simulink model "Boomerang_CoM_simulink"  (R2023a)
settings: Solver=ode4  StartTime=0.0  StopTime=t  FixedStep=dt  MaxStep=maxstep  MinStep=minstep
values from neighbouring files (symbols this model uses):
  c = 5e-2    (= 0.05)    [Boomerang4w_control.m]    (also in Boomerang_control_CoM.m = 0.0488; Boomerang_control_dihedral.m = 0.0488; Boomerang_control_gamma.m = 0.0488; Boomerang_control_pitch.m = 0.0488)
  CDdata = [x_CD, y_CD]    [Boomerang4w_control.m]    (also in Boomerang_control_CoM.m; Boomerang_control_dihedral.m; Boomerang_control_gamma.m; Boomerang_control_pitch.m)
  CLdata = [x_CL, y_CL]    [Boomerang4w_control.m]    (also in Boomerang_control_CoM.m; Boomerang_control_dihedral.m; Boomerang_control_gamma.m; Boomerang_control_pitch.m)
  CMdata = [x_CM, y_CM]    [Boomerang4w_control.m]    (also in Boomerang_control_CoM.m; Boomerang_control_dihedral.m; Boomerang_control_gamma.m; Boomerang_control_pitch.m)
  CoM_sat = 4e-2    (= 0.04)    [Boomerang4w_control.m]    (also in Boomerang_control_CoM.m = 0.02)
  Eul0 = [0; 0; 0]    [Boomerang4w_control.m]    (also in Boomerang_control_CoM.m; Boomerang_control_dihedral.m; Boomerang_control_gamma.m; Boomerang_control_pitch.m)
  g = 9.81    [Boomerang4w_control.m]    (also in Boomerang_control_CoM.m; Boomerang_control_dihedral.m; Boomerang_control_gamma.m; Boomerang_control_pitch.m)
  invTI0 = transpose(TI0)    [Boomerang4w_control.m]    (also in Boomerang_control_CoM.m; Boomerang_control_dihedral.m; Boomerang_control_gamma.m; Boomerang_control_pitch.m)
  J = J + (Ji(:,:,i))    [Boomerang4w_control.m]    (also in Boomerang_control_CoM.m = diag(diag(J)); Boomerang_control_dihedral.m = diag(diag(J)); Boomerang_control_gamma.m = diag(diag(J)); Boomerang_control_pitch.m = diag(diag(J)))
  Kd = 0.    (= 0)    [Boomerang4w_control.m]    (also in Boomerang_control_CoM.m; Boomerang_control_dihedral.m; Boomerang_control_gamma.m; Boomerang_control_pitch.m)
  Ki = 0.    (= 0)    [Boomerang4w_control.m]    (also in Boomerang_control_CoM.m; Boomerang_control_dihedral.m; Boomerang_control_gamma.m; Boomerang_control_pitch.m)
  Kp = .0    (= 0)    [Boomerang4w_control.m]    (also in Boomerang_control_CoM.m; Boomerang_control_dihedral.m; Boomerang_control_gamma.m; Boomerang_control_pitch.m)
  l_integrate = linspace(0,l_blade,n)    [Boomerang4w_control.m]    (also in Boomerang_control_CoM.m; Boomerang_control_dihedral.m; Boomerang_control_gamma.m; Boomerang_control_pitch.m)
  m = 200e-3    (= 0.2)    [Boomerang4w_control.m]    (also in Boomerang_control_CoM.m = 0.13; Boomerang_control_dihedral.m = 0.13; Boomerang_control_gamma.m = 0.13; Boomerang_control_pitch.m = 0.13)
  n = n + 1    (= 51)    [Boomerang4w_control.m]    (also in Boomerang_control_CoM.m; Boomerang_control_dihedral.m; Boomerang_control_gamma.m; Boomerang_control_pitch.m)
  nw = 4    [Boomerang4w_control.m]    (also in Boomerang_control_CoM.m = 2; Boomerang_control_dihedral.m = 2; Boomerang_control_gamma.m = 2; Boomerang_control_pitch.m = 2)
  omega0 = [0; 0; 10*pi*2]    [Boomerang4w_control.m]    (also in Boomerang_control_CoM.m; Boomerang_control_dihedral.m; Boomerang_control_gamma.m; Boomerang_control_pitch.m)
  PHI0 = deg2rad(PHI0)    [Boomerang4w_control.m]    (also in Boomerang_control_CoM.m; Boomerang_control_dihedral.m; Boomerang_control_gamma.m; Boomerang_control_pitch.m)
  PSI0 = deg2rad(PSI0)    [Boomerang4w_control.m]    (also in Boomerang_control_CoM.m; Boomerang_control_dihedral.m; Boomerang_control_gamma.m; Boomerang_control_pitch.m)
  R_pos0 = [0; 0; 1.5]    [Boomerang4w_control.m]    (also in Boomerang_control_CoM.m; Boomerang_control_dihedral.m; Boomerang_control_gamma.m; Boomerang_control_pitch.m)
  rate = 1    [Boomerang4w_control.m]    (also in Boomerang_control_CoM.m)
  rho = 1.22    [Boomerang4w_control.m]    (also in Boomerang_control_CoM.m; Boomerang_control_dihedral.m; Boomerang_control_gamma.m; Boomerang_control_pitch.m)
  S = pi*R^2    (= 0.196349540849)    [Boomerang4w_control.m]    (also in Boomerang_control_CoM.m = 0.228; Boomerang_control_dihedral.m = 0.228; Boomerang_control_gamma.m = 0.228; Boomerang_control_pitch.m = 0.228)
  THETA0 = deg2rad(THETA0)    [Boomerang4w_control.m]    (also in Boomerang_control_CoM.m; Boomerang_control_dihedral.m; Boomerang_control_gamma.m; Boomerang_control_pitch.m)
  thetaj = 25    [Boomerang4w_control.m]    (also in Boomerang_control_CoM.m = deg2rad(thetaj); Boomerang_control_dihedral.m = deg2rad(thetaj); Boomerang_control_gamma.m = deg2rad(thetaj); Boomerang_control_pitch.m = deg2rad(thetaj))
  TI0 = RI01*RI02*RI03    [Boomerang4w_control.m]    (also in Boomerang_control_CoM.m; Boomerang_control_dihedral.m; Boomerang_control_gamma.m; Boomerang_control_pitch.m)
  u0 = TI0*U0    [Boomerang4w_control.m]    (also in Boomerang_control_CoM.m; Boomerang_control_dihedral.m; Boomerang_control_gamma.m; Boomerang_control_pitch.m)
  v_wind = [-1; 0; 0]    [Boomerang4w_control.m]    (also in Boomerang_control_CoM.m = [0; 0; 0]; Boomerang_control_dihedral.m = [0; 0; 0]; Boomerang_control_gamma.m = [0; 0; 0]; Boomerang_control_pitch.m = [0; 0; 0])
  x_ac = zeros(3,nw)    [Boomerang4w_control.m]    (also in Boomerang_control_CoM.m = 0.061; Boomerang_control_dihedral.m = 0.061; Boomerang_control_gamma.m = 0.061; Boomerang_control_pitch.m = 0.061)
  X_des = [x_des, y_des]    [Boomerang4w_control.m]    (also in Boomerang_control_CoM.m; Boomerang_control_dihedral.m; Boomerang_control_gamma.m; Boomerang_control_pitch.m)
libraries: simulink_extras x1
settings Model: Creator=dsantis  LastModifiedBy=dsantis

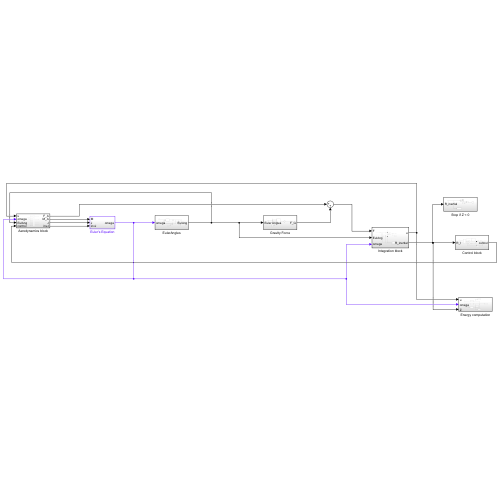
[thumbnail: Simulink's stored preview of the top-level diagram]
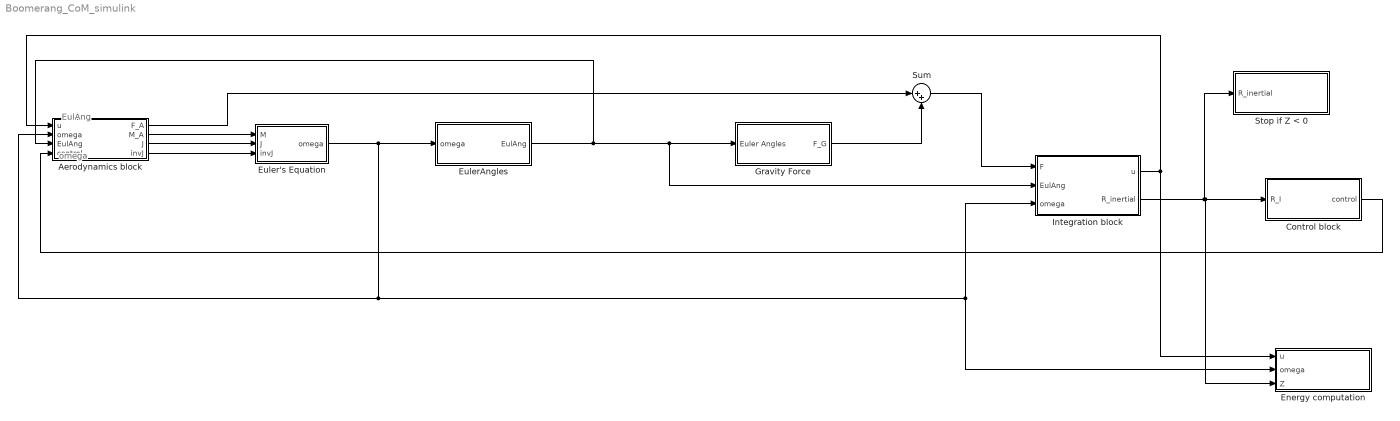
== system Boomerang_CoM_simulink ==
  note: omega
  note: EulAng
  Aerodynamics block : Subsystem
  Control block : Subsystem
  Energy computation : Subsystem
  Euler's Equation : Subsystem
  EulerAngles : Subsystem
  Gravity Force : Subsystem
  Integration block : Subsystem
  Stop if Z < 0 : Subsystem
  Sum : Sum  Inputs=|++
  wires:
  Sum/1 -> Integration block/1(F)
  Aerodynamics block/2(M_A) -> Euler's Equation/1(M)
  Aerodynamics block/1(F_A) -> Sum/1
  Integration block/1(u) -> Energy computation/1(u), Aerodynamics block/1(u)
  Aerodynamics block/4(invJ) -> Euler's Equation/3(invJ)
  Aerodynamics block/3(J) -> Euler's Equation/2(J)
  Integration block/2(R_inertial) -> Energy computation/3(Z), Control block/1(R_I), Stop if Z < 0/1(R_inertial)
  EulerAngles/1(EulAng) -> Integration block/2(EulAng), Gravity Force/1(Euler Angles), Aerodynamics block/3(EulAng)
  Euler's Equation/1(omega) -> Aerodynamics block/2(omega), Energy computation/2(omega), Integration block/3(omega), EulerAngles/1(omega)
  Gravity Force/1(F_G) -> Sum/2
  Control block/1(control) -> Aerodynamics block/4(control)

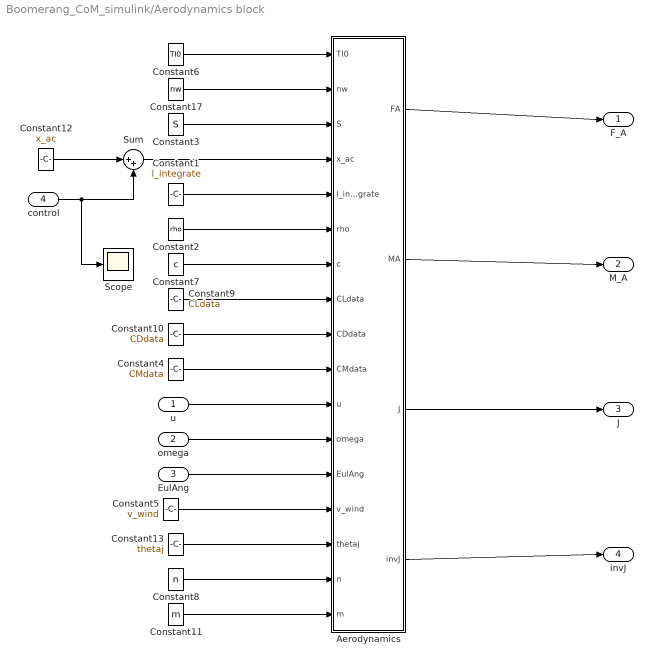
== system Boomerang_CoM_simulink/Aerodynamics block ==
  u : Inport
  omega : Inport  Port=2
  EulAng : Inport  Port=3
  control : Inport  Port=4
  Aerodynamics : MATLAB Function  TreatAsAtomicUnit=on
  Constant1 : Constant  Value=l_integrate
  Constant10 : Constant  Value=CDdata
  Constant11 : Constant  Value=m
  Constant12 : Constant  Value=x_ac
  Constant13 : Constant  Value=thetaj
  Constant17 : Constant  Value=nw
  Constant2 : Constant  Value=rho
  Constant3 : Constant  Value=S
  Constant4 : Constant  Value=CMdata
  Constant5 : Constant  Value=v_wind
  Constant6 : Constant  Value=TI0
  Constant7 : Constant  Value=c
  Constant8 : Constant  Value=n
  Constant9 : Constant  Value=CLdata
  Scope : Scope
  Sum : Sum  Inputs=|++
  F_A : Outport
  M_A : Outport  Port=2
  J : Outport  Port=3
  invJ : Outport  Port=4
  wires:
  u/1 -> Aerodynamics/11(u)
  Constant2/1 -> Aerodynamics/6(rho)
  Constant9/1 -> Aerodynamics/8(CLdata)
  Constant10/1 -> Aerodynamics/9(CDdata)
  Constant1/1 -> Aerodynamics/5(l_integrate)
  Constant7/1 -> Aerodynamics/7(c)
  omega/1 -> Aerodynamics/12(omega)
  Constant12/1 -> Sum/1
  Constant17/1 -> Aerodynamics/2(nw)
  Constant3/1 -> Aerodynamics/3(S)
  Aerodynamics/1(FA) -> F_A/1
  Constant4/1 -> Aerodynamics/10(CMdata)
  Aerodynamics/2(MA) -> M_A/1
  EulAng/1 -> Aerodynamics/13(EulAng)
  Constant5/1 -> Aerodynamics/14(v_wind)
  Constant6/1 -> Aerodynamics/1(TI0)
  Constant8/1 -> Aerodynamics/16(n)
  Aerodynamics/3(J) -> J/1
  Aerodynamics/4(invJ) -> invJ/1
  Constant11/1 -> Aerodynamics/17(m)
  Constant13/1 -> Aerodynamics/15(thetaj)
  control/1 -> Scope/1, Sum/2
  Sum/1 -> Aerodynamics/4(x_ac)

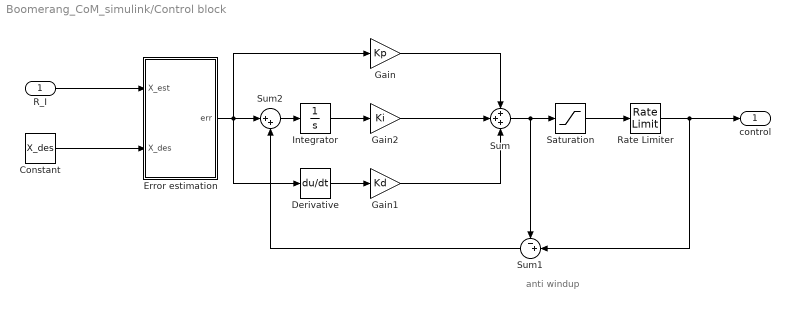
== system Boomerang_CoM_simulink/Control block ==
  note: anti windup
  R_I : Inport
  Constant : Constant  Value=X_des
  Derivative : Derivative
  Error estimation : MATLAB Function  TreatAsAtomicUnit=on
  Gain : Gain  Gain=Kp
  Gain1 : Gain  Gain=Kd
  Gain2 : Gain  Gain=Ki
  Integrator : Integrator  UpperSaturationLimit=pi/Ki  LowerSaturationLimit=-pi/Ki
  Rate Limiter : RateLimiter  RisingSlewLimit=rate  FallingSlewLimit=-rate  SampleTimeMode=inherited
  Saturation : Saturate  UpperLimit=CoM_sat  LowerLimit=-CoM_sat
  Sum : Sum  Inputs=+++
  Sum1 : Sum  Inputs=-+|
  Sum2 : Sum  Inputs=|++
  control : Outport
  wires:
  R_I/1 -> Error estimation/1(X_est)
  Constant/1 -> Error estimation/2(X_des)
  Error estimation/1(err) -> Sum2/1, Derivative/1, Gain/1
  Gain/1 -> Sum/1
  Derivative/1 -> Gain1/1
  Gain1/1 -> Sum/3
  Saturation/1 -> Rate Limiter/1
  Rate Limiter/1 -> Sum1/2, control/1
  Integrator/1 -> Gain2/1
  Gain2/1 -> Sum/2
  Sum2/1 -> Integrator/1
  Sum1/1 -> Sum2/2
  Sum/1 -> Saturation/1, Sum1/1

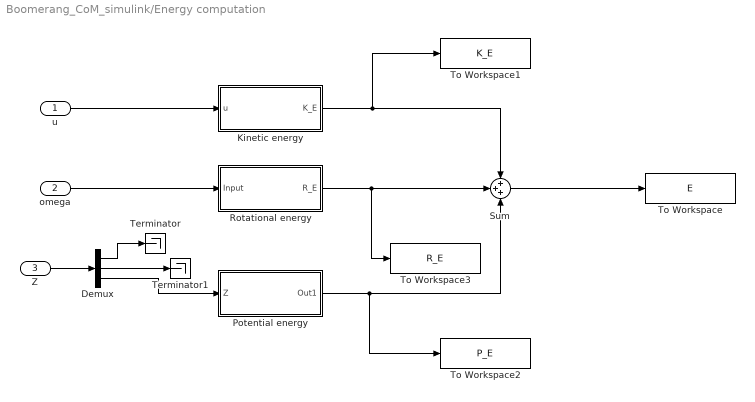
== system Boomerang_CoM_simulink/Energy computation ==
  u : Inport
  omega : Inport  Port=2
  Z : Inport  Port=3
  Demux : Demux  Outputs=3
  Kinetic energy : Subsystem
  Potential energy : Subsystem
  Rotational energy : Subsystem
  Sum : Sum  Inputs=+++
  Terminator : Terminator
  Terminator1 : Terminator
  To Workspace : ToWorkspace  VariableName=E  SaveFormat=Timeseries  SampleTime=-1
  To Workspace1 : ToWorkspace  VariableName=K_E  SaveFormat=Timeseries  SampleTime=-1
  To Workspace2 : ToWorkspace  VariableName=P_E  SaveFormat=Timeseries  SampleTime=-1
  To Workspace3 : ToWorkspace  VariableName=R_E  SaveFormat=Timeseries  SampleTime=-1
  wires:
  u/1 -> Kinetic energy/1(u)
  omega/1 -> Rotational energy/1(Input)
  Z/1 -> Demux/1
  Demux/3 -> Potential energy/1(Z)
  Demux/1 -> Terminator/1
  Demux/2 -> Terminator1/1
  Kinetic energy/1(K_E) -> To Workspace1/1, Sum/1
  Rotational energy/1(R_E) -> To Workspace3/1, Sum/2
  Potential energy/1(Out1) -> To Workspace2/1, Sum/3
  Sum/1 -> To Workspace/1

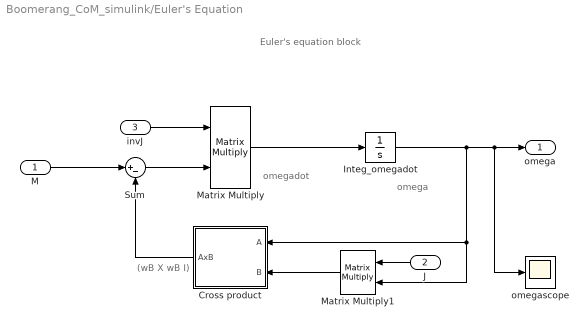
== system Boomerang_CoM_simulink/Euler's Equation ==
  note: Euler's equation block
  note: (wB X wB I)
  note: omega
  note: omegadot
  M : Inport
  J : Inport  Port=2
  invJ : Inport  Port=3
  Cross product : Subsystem
  Integ_omegadot : Integrator  InitialCondition=omega0
  Matrix Multiply : Product  Multiplication=Matrix(*)
  Matrix Multiply1 : Product  Multiplication=Matrix(*)
  Sum : Sum  Inputs=|+-
  omegascope : Scope
  omega : Outport  VectorParamsAs1DForOutWhenUnconnected=off
  wires:
  Integ_omegadot/1 -> Cross product/1(A), Matrix Multiply1/2, omegascope/1, omega/1
  Matrix Multiply1/1 -> Cross product/2(B)
  M/1 -> Sum/1
  Sum/1 -> Matrix Multiply/2
  Matrix Multiply/1 -> Integ_omegadot/1
  Cross product/1(AxB) -> Sum/2
  invJ/1 -> Matrix Multiply/1
  J/1 -> Matrix Multiply1/1

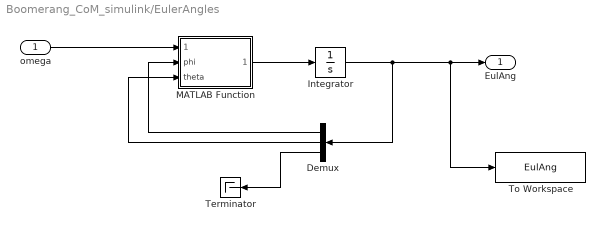
== system Boomerang_CoM_simulink/EulerAngles ==
  omega : Inport
  Demux : Demux  Outputs=3
  Integrator : Integrator  InitialCondition=Eul0
  MATLAB Function : MATLAB Function  TreatAsAtomicUnit=on
  Terminator : Terminator
  To Workspace : ToWorkspace  VariableName=EulAng  SampleTime=-1
  EulAng : Outport
  wires:
  omega/1 -> MATLAB Function/1(omega)
  MATLAB Function/1(EulRate) -> Integrator/1
  Integrator/1 -> Demux/1, To Workspace/1, EulAng/1
  Demux/1 -> MATLAB Function/2(phi)
  Demux/2 -> MATLAB Function/3(theta)
  Demux/3 -> Terminator/1

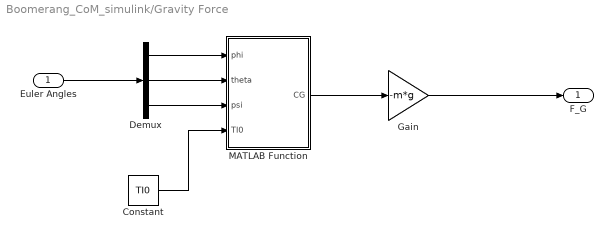
== system Boomerang_CoM_simulink/Gravity Force ==
  Euler Angles : Inport
  Constant : Constant  Value=TI0
  Demux : Demux  Outputs=3
  Gain : Gain  Gain=-m*g
  MATLAB Function : MATLAB Function  TreatAsAtomicUnit=on
  F_G : Outport
  wires:
  Gain/1 -> F_G/1
  Demux/3 -> MATLAB Function/3(psi)
  Demux/2 -> MATLAB Function/2(theta)
  Demux/1 -> MATLAB Function/1(phi)
  MATLAB Function/1(CG) -> Gain/1
  Euler Angles/1 -> Demux/1
  Constant/1 -> MATLAB Function/4(TI0)

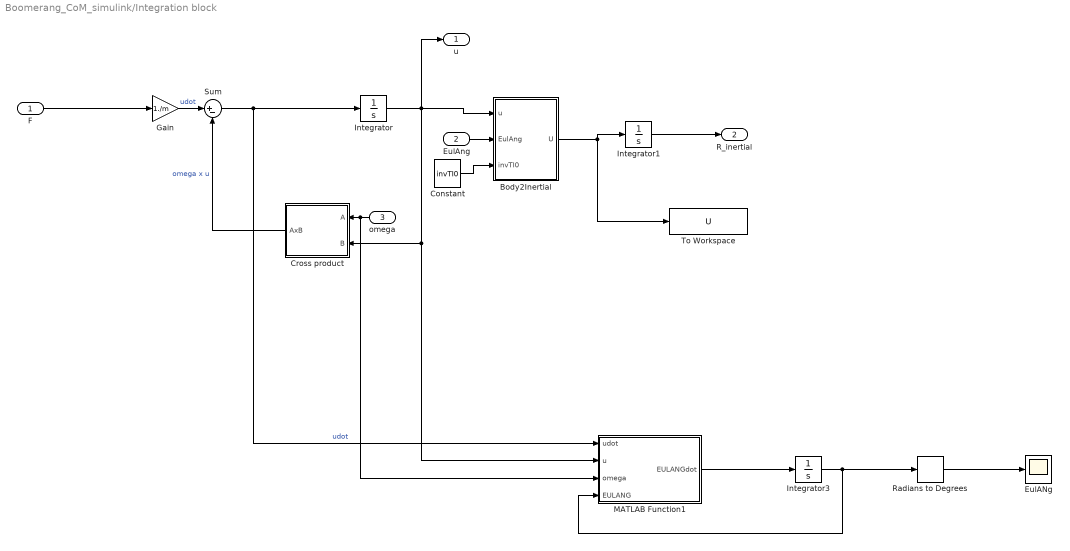
== system Boomerang_CoM_simulink/Integration block ==
  F : Inport
  EulAng : Inport  Port=2
  omega : Inport  Port=3
  Body2Inertial : MATLAB Function  TreatAsAtomicUnit=on
  Constant : Constant  Value=invTI0
  Cross product : Subsystem
  EulANg : Scope
  Gain : Gain  Gain=1./m
  Integrator : Integrator  InitialCondition=u0
  Integrator1 : Integrator  InitialCondition=R_pos0
  Integrator3 : Integrator  InitialCondition=[PHI0; THETA0; PSI0]
  MATLAB Function1 : MATLAB Function  TreatAsAtomicUnit=on
  Radians to Degrees : simulink_extras/Transformations/Radians to Degrees
  Sum : Sum  Inputs=|+-
  To Workspace : ToWorkspace  VariableName=U  SampleTime=-1
  u : Outport
  R_inertial : Outport  Port=2
  wires:
  Cross product/1(AxB) -> Sum/2  "omega x u"
  Integrator/1 -> MATLAB Function1/2(u), Cross product/2(B), Body2Inertial/1(u), u/1
  Integrator1/1 -> R_inertial/1
  Gain/1 -> Sum/1  "udot"
  EulAng/1 -> Body2Inertial/2(EulAng)
  Constant/1 -> Body2Inertial/3(invTI0)
  F/1 -> Gain/1
  Body2Inertial/1(U) -> Integrator1/1, To Workspace/1
  Sum/1 -> MATLAB Function1/1(udot), Integrator/1  "udot"
  omega/1 -> MATLAB Function1/3(omega), Cross product/1(A)
  MATLAB Function1/1(EULANGdot) -> Integrator3/1
  Integrator3/1 -> Radians to Degrees/1, MATLAB Function1/4(EULANG)
  Radians to Degrees/1 -> EulANg/1

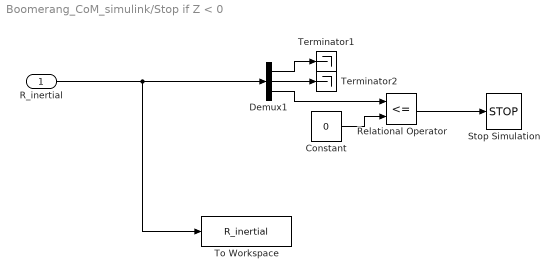
== system Boomerang_CoM_simulink/Stop if Z < 0 ==
  R_inertial : Inport
  Constant : Constant  Value=0
  Demux1 : Demux  Outputs=3
  Relational Operator : RelationalOperator  Operator=<=  OutDataTypeStr=boolean  RndMeth=Simplest  InputSameDT=off
  Stop Simulation : Stop
  Terminator1 : Terminator
  Terminator2 : Terminator
  To Workspace : ToWorkspace  VariableName=R_inertial  SampleTime=-1
  wires:
  R_inertial/1 -> To Workspace/1, Demux1/1
  Demux1/1 -> Terminator1/1
  Demux1/3 -> Relational Operator/1
  Demux1/2 -> Terminator2/1
  Constant/1 -> Relational Operator/2
  Relational Operator/1 -> Stop Simulation/1

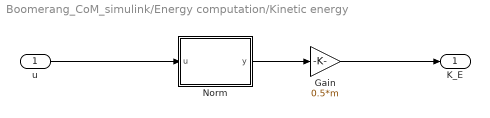
== system Boomerang_CoM_simulink/Energy computation/Kinetic energy ==
  u : Inport
  Gain : Gain  Gain=0.5*m
  Norm : MATLAB Function  TreatAsAtomicUnit=on
  K_E : Outport
  wires:
  u/1 -> Norm/1(u)
  Norm/1(y) -> Gain/1
  Gain/1 -> K_E/1

== system Boomerang_CoM_simulink/Energy computation/Potential energy ==
  Z : Inport
  Gain : Gain  Gain=m*g
  Out1 : Outport
  wires:
  Z/1 -> Gain/1
  Gain/1 -> Out1/1

== system Boomerang_CoM_simulink/Energy computation/Rotational energy ==
  Input : Inport
  Dot Product : DotProduct  OutDataTypeStr=Inherit: Inherit via internal rule
  Gain : Gain  Gain=0.5*J  Multiplication=Matrix(u*K)
  R_E : Outport
  wires:
  Input/1 -> Dot Product/2, Gain/1
  Gain/1 -> Dot Product/1
  Dot Product/1 -> R_E/1

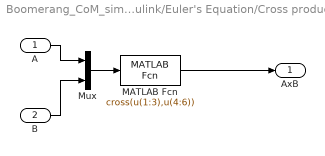
== system Boomerang_CoM_simulink/Euler's Equation/Cross product ==
  A : Inport
  B : Inport  Port=2
  MATLAB Fcn : MATLABFcn  MATLABFcn=cross(u(1:3),u(4:6))
  Mux : Mux  Inputs=2
  AxB : Outport  VectorParamsAs1DForOutWhenUnconnected=off
  wires:
  A/1 -> Mux/1
  B/1 -> Mux/2
  Mux/1 -> MATLAB Fcn/1
  MATLAB Fcn/1 -> AxB/1

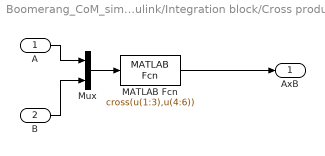
== system Boomerang_CoM_simulink/Integration block/Cross product ==
  A : Inport
  B : Inport  Port=2
  MATLAB Fcn : MATLABFcn  MATLABFcn=cross(u(1:3),u(4:6))
  Mux : Mux  Inputs=2
  AxB : Outport  VectorParamsAs1DForOutWhenUnconnected=off
  wires:
  A/1 -> Mux/1
  B/1 -> Mux/2
  Mux/1 -> MATLAB Fcn/1
  MATLAB Fcn/1 -> AxB/1

== matlab function Boomerang_CoM_simulink/Energy computation/Kinetic energy/Norm ==
  data: u input; y output
function y = fcn(u)

y = norm(u)^2;

== matlab function Boomerang_CoM_simulink/Integration block/MATLAB Function1 ==
  data: udot input; u input; EULANGdot output; omega input; EULANG input
function EULANGdot = fcn(udot, u, omega, EULANG)
udotx = udot(1);
udoty = udot(2);

ux = u(1);
uy = u(2);

p = omega(1);
q = omega(2);
r = omega(3);

PHI = EULANG(1);
THETA = EULANG(2);

rn = r + (udoty*ux - udotx*uy)/(ux^2 + uy^2);
lambda = -tan(uy/ux);

PHIdot = (p*cos(lambda) - q*sin(lambda)) + (p*sin(lambda) + q*cos(lambda))*sin(PHI)*tan(THETA) + ...
    rn*cos(PHI)*tan(THETA);
THETAdot = (p*sin(lambda) + q*cos(lambda))*cos(PHI) - rn*sin(PHI);
PSIdot = (p*sin(lambda) + q*cos(lambda))*sin(PHI)/cos(THETA) + rn*cos(PHI)/cos(THETA);

EULANGdot = [PHIdot; THETAdot; PSIdot];

== matlab function Boomerang_CoM_simulink/Aerodynamics block/Aerodynamics ==
  settings: updateMethod=DISCRETE
  data: TI0 input; nw input; S input; x_ac input; l_integrate input; rho input; c input; CLdata input; CDdata input; CMdata input; u input; omega input; EulAng input; v_wind input; FA output; thetaj input; MA output; n input; J output; invJ output; m input
function [FA, MA, J, invJ] = fcn(TI0, nw, S, x_ac, l_integrate, rho, c, CLdata, CDdata, CMdata,u, omega, EulAng, v_wind, thetaj, n, m)
phi = EulAng(1);
theta = EulAng(2);
psi = EulAng(3);

R01 = [1, 0, 0; 0, cos(phi), sin(phi); 0, -sin(phi), cos(phi)];
R02 = [cos(theta), 0, -sin(theta); 0, 1, 0; sin(theta), 0, cos(theta)];
R03 = [cos(psi), sin(psi), 0; -sin(psi), cos(psi), 0; 0, 0, 1];
T0 = R01*R02*R03;

Tj = zeros(3,3, nw);
invTj = zeros(3,3,nw);

I_xi = 1.88e-3; 
I_eta = 4.88e-6;
I_zeta = 1.92e-3;
I_xieta = 5.14e-21;

LAMBDAj = 120;  % Wing sweep angle [deg]
LAMBDAj = deg2rad(LAMBDAj);
gamma = 120;    % Folding angle [deg]
gamma = deg2rad(gamma);
betaj = 0;      % Wing coning angle 
betaj = deg2rad(betaj);

Jj = [
    I_xi I_xieta 0;
    I_xieta I_eta 0;
    0 0 I_zeta
    ];

for i = 0:(nw-1)
Rj1 = [1, 0, 0; 0, cos(betaj), sin(betaj); 0, -sin(betaj), cos(betaj)];
    Rj2 = [cos(thetaj), 0, -sin(thetaj);0, 1, 0; sin(thetaj), 0, cos(thetaj)];
    Rj3 = [cos(LAMBDAj-pi/2 + gamma*i), sin(LAMBDAj-pi/2 + gamma*i), 0; ...
        -sin(LAMBDAj-pi/2 + gamma*i), cos(LAMBDAj-pi/2+ gamma*i), 0;0, 0, 1];
    Tj(:,:,i+1) = Rj2*Rj1*Rj3;
    invTj(:,:,i+1) = transpose(Tj(:,:,i+1));
end
Ji = zeros(3,3,nw);
J = zeros(3);
for i = 1:nw
    Ji(:,:,i) = invTj(:,:,i)*Jj*Tj(:,:,i);
    J = J + (Ji(:,:,i));
end

J(2,2) = J(2,2) + m*x_ac^2;
J(3,3) = J(3,3) + m*x_ac^2;

J = diag(diag(J));

invJ = inv(J);

persistent flag FAz
if isempty(flag)
    flag = false;
    FAz = 0;
end

f = @(v_ind) v_ind - FAz/(2*rho*S*sqrt(u(1)^2 + (u(3)-v_ind)^2));
v_ind = fzero(f,0);

v_ind = [0; 0; -v_ind];
% Piecewise linear fit for CL
C_L = @(alpha) interp1(CLdata(:,1), CLdata(:,2), alpha, 'linear', 'extrap');

% Piecewise linear fit for CD
C_D = @(alpha) interp1(CDdata(:,1), CDdata(:,2), alpha, 'linear', 'extrap');

 % Piecewise linear fit for CM
C_M = @(alpha) interp1(CMdata(:,1), CMdata(:,2), alpha, 'linear', 'extrap');

FA = [0; 0; 0];
MA = [0;0;0];

for i = 1:nw
    rA = [x_ac.*ones(1,n); zeros(1,n); zeros(1,n)] + invTj(:,:,i)*[zeros(1,n); l_integrate'; zeros(1,n)];
    
    w = Tj(:,:,i)*( (-u -cross(omega.*ones(3,n), rA)) - v_ind + T0*TI0*v_wind);
    alpha = atan2(w(3,:),w(1,:)) + thetaj;

    w2 = w(1,:).^2 + w(3,:).^2;

    l = (0.5*rho*c).*w2.*C_L(alpha);
    d = (0.5*rho*c).*w2.*C_D(alpha);
    m_eta = (0.5*rho*c^2).*w2.*C_M(alpha);

    int_funx = -l.*sin(alpha) + d.*cos(alpha);
    int_funz = l.*cos(alpha) + d.*sin(alpha);
    int_funMx = (l.*cos(alpha) + d.*sin(alpha)).*l_integrate';
    int_funMy = m_eta; 
    int_funMz = (-l.*sin(alpha) + d.*cos(alpha)).*l_integrate';
 
    FxjA = trapz(l_integrate,int_funx);
    FzjA = trapz(l_integrate,int_funz);

    MxjA = trapz(l_integrate,int_funMx);
    MyjA = trapz(l_integrate,int_funMy);
    MzjA = trapz(l_integrate,int_funMz);

    FjA = [FxjA; 0; FzjA];
    FA = FA + invTj(:,:,i)*FjA;

    MjA = [MxjA; MyjA; MzjA];
    MA = MA + invTj(:,:,i)*MjA + cross([x_ac; 0; 0], invTj(:,:,i)*FjA);
    
end

FAz = FA(3);

== matlab function Boomerang_CoM_simulink/Gravity Force/MATLAB Function ==
  data: phi input; theta input; psi input; CG output; TI0 input
function CG = fcn(phi, theta, psi, TI0)
R01 = [
    1, 0, 0;
    0, cos(phi), sin(phi);
    0, -sin(phi), cos(phi)
    ];
R02 = [
    cos(theta), 0, -sin(theta);
    0, 1, 0;
    sin(theta), 0, cos(theta)
];
R03 = [
    cos(psi), sin(psi), 0;
    -sin(psi), cos(psi), 0;
    0, 0, 1
];
T0 = R01*R02*R03;

CG = T0*TI0*[0; 0; 1];

== matlab function Boomerang_CoM_simulink/Integration block/Body2Inertial ==
  data: u input; U output; EulAng input; invTI0 input
function U = fcn(u, EulAng, invTI0)
phi = EulAng(1);
theta = EulAng(2);
psi = EulAng(3);

R01 = [
    1, 0, 0;
    0, cos(phi), sin(phi);
    0, -sin(phi), cos(phi)
    ];
R02 = [
    cos(theta), 0, -sin(theta);
    0, 1, 0;
    sin(theta), 0, cos(theta)
];
R03 = [
    cos(psi), sin(psi), 0;
    -sin(psi), cos(psi), 0;
    0, 0, 1
];
T0 = R01*R02*R03;
invT0 = transpose(T0);
U = invTI0*invT0*u;

== matlab function Boomerang_CoM_simulink/EulerAngles/MATLAB Function ==
  data: omega input; EulRate output; phi input; theta input
function EulRate = fcn(omega, phi, theta)

phidot = omega(1) + omega(2)*sin(phi)*tan(theta) + omega(3)*cos(phi)*tan(theta);
thetadot = omega(2)*cos(phi) - omega(3)*sin(phi);
psidot = omega(2)*sin(phi)/cos(theta) + omega(3)*cos(phi)/cos(theta);

EulRate = [phidot; thetadot; psidot];

== matlab function Boomerang_CoM_simulink/Control block/Error estimation ==
  settings: updateMethod=DISCRETE
  data: X_est input; err output; X_des input
function err = fcn(X_est,X_des)

% Find which desired trajectory point is nearest to the boomerang and
% compute the error. 
[err_vec, i] = min(vecnorm([X_est(1), X_est(2)] - X_des,2,2));

% Figure out if you are to the left or to the right of the desired
% trajectory in order to determine the sign of the error and follow with
% the proper control maneuver
err_sign = sign(norm([X_est(1), X_est(2)]) - norm([X_des(i,1), X_des(i,2)]));

err = err_sign*err_vec;

end
